simulink model "lqr"  (R2017a)
settings: Solver=VariableStepAuto  StartTime=0.0  StopTime=25  RelTol=1e-3
values from neighbouring files (symbols this model uses):
  A = [-8.8487+(a-b)/5 -0.0399 -5.55+(c+d)/10 3.5846 ... (first row only)    [initialize.m]
  B = [0.0564+b/(10+c) 0.0319 ... (first row only)    [initialize.m]
  C = [-3.2988 -2.1932+(10*c+d)/(100+5*a) 0.037 -0.0109 ... (first row only)    [initialize.m]
  K_LQR = real(K_LQR)    [LQR.m]    (also in MIMO_servo_control_with_observer.m; MIMO_servo_control_without_observer.m; full_order_observer.m; last_task.m)
settings Model: Creator=lenovo  LastModifiedBy=lenovo

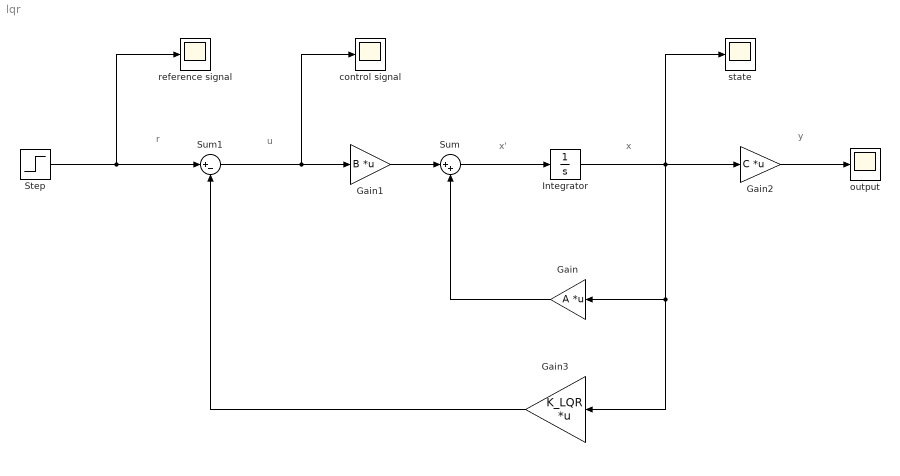
== system lqr ==
  note: x'
  note: x
  note: y
  note: u
  note: r
  Gain : Gain  Gain=A  Multiplication=Matrix(K*u)
  Gain1 : Gain  Gain=B  Multiplication=Matrix(K*u)
  Gain2 : Gain  Gain=C  Multiplication=Matrix(K*u)
  Gain3 : Gain  Gain=K_LQR  Multiplication=Matrix(K*u)
  Integrator : Integrator  InitialCondition=[0.5;-0.1;0.3;-0.8]
  Step : Step  Time=0  Before=[0;0]  After=[0;0]  SampleTime=0  VectorParams1D=off
  Sum : Sum  Inputs=|++
  Sum1 : Sum  Inputs=|+-
  control signal : Scope
  output : Scope
  reference signal : Scope
  state : Scope
  wires:
  Gain/1 -> Sum/2
  Integrator/1 -> Gain3/1, Gain/1, Gain2/1, state/1
  Step/1 -> reference signal/1, Sum1/1
  Sum1/1 -> control signal/1, Gain1/1
  Gain2/1 -> output/1
  Gain3/1 -> Sum1/2
  Sum/1 -> Integrator/1
  Gain1/1 -> Sum/1
